simulink model "homework4"  (R2015a)
settings: Solver=ode45  StartTime=0.0  StopTime=15  RelTol=1e-3
values from neighbouring files (symbols this model uses):
  A = [[X_u, X_w, 0, -g*cos(theta_0)] ... (first row only)    [hw4.m]
  B = [-(X_u)                             -(X_w)                             X_d_e ... (first row only)    [hw4.m]
  C = [1 0     0 0 ... (first row only)    [hw4.m]
  D = [0 0 0 ... (first row only)    [hw4.m]
  u_0 = 634    [hw4.m]
undefined symbols (not defined in the file or in its folder): sigbuilder_block
settings Model: Creator=rjoyce  LastModifiedBy=karasinski
settings DataIOCC: SignalLoggingSaveFormat=ModelDataLogs
settings OptimizationCC: ExpressionDepthLimit=2147483647
settings DebuggingCC: UnderspecifiedInitializationDetection=Classic  MergeDetectMultiDrivingBlocksExec=none  SolverPrmCheckMsg=warning  FcnCallInpInsideContextMsg=UseLocalSettings  StateNameClashWarn=warning
settings GRTTargetCC: CombineOutputUpdateFcns=off  GRTInterface=on

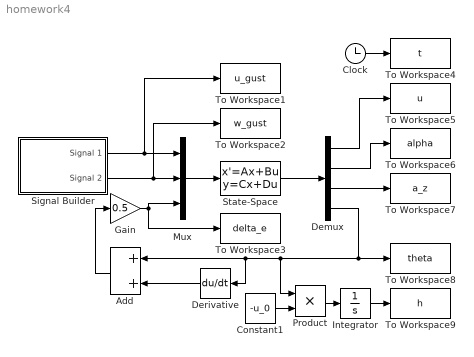
== system homework4 ==
  Add : Sum
  Clock : Clock
  Constant1 : Constant  Value=-u_0
  Demux : Demux
  Derivative : Derivative
  Gain : Gain  Gain=0.5
  Integrator : Integrator
  Mux : Mux  Inputs=3
  Product : Product
  Signal Builder : Subsystem  Tag=STV Subsys  LoadFcn=sigbuilder_block('load');  StartFcn=sigbuilder_block('start');  StopFcn=sigbuilder_block('stop');  ClipboardFcn=sigbuilder_block('clipboard');  mask(Sigbuilder block){}
      mask help: Simulink:masks:SigbuilderBlock_MD
      mask init:
      | if ~strcmp(get_param(bdroot(gcbh),'SimulationStatus'),'stopped') tuvar = sigbuilder_block('maskInit'); end
      settings: CopyFcn=sigbuilder_block('copy');  DeleteFcn=sigbuilder_block('delete');  ModelCloseFcn=sigbuilder_block('modelClose');  PreSaveFcn=sigbuilder_block('preSave');  PauseFcn=sigbuilder_block('pause');  ContinueFcn=sigbuilder_block('continue');  NameChangeFcn=sigbuilder_block('namechange');  OpenFcn=sigbuilder_block('open',[437.6 199.2 550.4 400 ]);  CloseFcn=sigbuilder_block('close');
      mask Display: plot(0, 0, 100, 100,[2, 2, 32, 32, 2], [68, 8, 8, 68, 68],[32, 2], [38, 38], [32, 19, 2],[53, 60, 44], [32, 17, 17, 2],[16, 16, 31, 31]);txt = getActiveGroup(gcbh);text(2, 100, txt,'verticalAlignment', 'top');
  State-Space : StateSpace  A=A  B=B  C=C  D=D  X0=0
  To Workspace1 : ToWorkspace  VariableName=u_gust  SampleTime=-1
  To Workspace2 : ToWorkspace  VariableName=w_gust  SampleTime=-1
  To Workspace3 : ToWorkspace  VariableName=delta_e  SampleTime=-1
  To Workspace4 : ToWorkspace  VariableName=t  SampleTime=-1
  To Workspace5 : ToWorkspace  VariableName=u  SampleTime=-1
  To Workspace6 : ToWorkspace  VariableName=alpha  SampleTime=-1
  To Workspace7 : ToWorkspace  VariableName=a_z  SampleTime=-1
  To Workspace8 : ToWorkspace  VariableName=theta  SampleTime=-1
  To Workspace9 : ToWorkspace  VariableName=h  SampleTime=-1
  wires:
  State-Space/1 -> Demux/1
  Mux/1 -> State-Space/1
  Demux/1 -> To Workspace5/1
  Demux/2 -> To Workspace6/1
  Gain/1 -> To Workspace3/1, Mux/3
  Clock/1 -> To Workspace4/1
  Signal Builder/1(Signal 1) -> To Workspace1/1, Mux/1
  Signal Builder/2(Signal 2) -> To Workspace2/1, Mux/2
  Product/1 -> Integrator/1
  Constant1/1 -> Product/2
  Integrator/1 -> To Workspace9/1
  Demux/3 -> To Workspace7/1
  Derivative/1 -> Add/2
  Add/1 -> Gain/1
  Demux/4 -> Derivative/1, Add/1, Product/1, To Workspace8/1

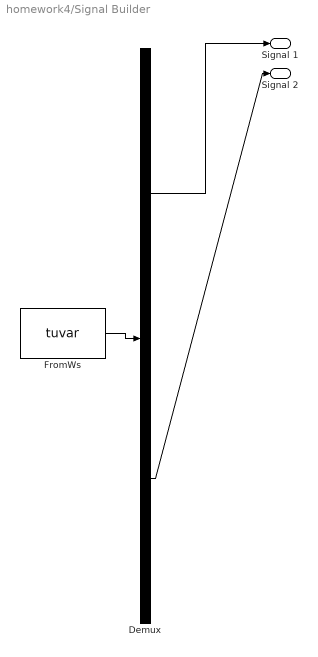
== system homework4/Signal Builder ==
  Demux : Demux  Tag=STV Demux  Outputs=2
  FromWs : FromWorkspace  Tag=STV FromWs  VariableName=tuvar  SampleTime=0
      SigBuilderData=|
      | common.afterFinalStr = 'Extrapolate'
      | common.sampleTime = 0
      | dataSet.timeRange = [0 15]
      | dataSet.name = 'Group 1'
      | sbobj.Groups.Name = 'Group 1'
      | sbobj.Groups.Signals(1).Name = 'Signal 1'
      | sbobj.Groups.Signals(1).XData = [0 1.5773 4.7319 6.3091 15]
      | sbobj.Groups.Signals(1).YData = [0 100 100 0 0]
      | sbobj.Groups.Signals(2).Name = 'Signal 2'
      | sbobj.Groups.Signals(2).XData = [0 3.1546 6.3091 15]
      | sbobj.Groups.Signals(2).YData = [0 -100 0 0]
      | sbobj.Groups.TimeRange = [0 15]
  Signal 1 : Outport  Tag=STV Outport
  Signal 2 : Outport  Tag=STV Outport  Port=2
  wires:
  Demux/1 -> Signal 1/1
  FromWs/1 -> Demux/1
  Demux/2 -> Signal 2/1
